simulink model "PMSM_FOC34"  (R2020b)
settings: Solver=FixedStepAuto  StartTime=0.0  StopTime=0.5  RelTol=1e-3
InitFcn:
  | Phi = 0.1;
  | Ld = 0.01;
  | Lq = 0.02;
  | Rs = 0.38;
  | p = 2;
  | Jm = 0.1e-3;
  | Dm = 1e-3;
  | Vdc = 100;
  | fc = 10e3;
  | Ts = 1/fc/100;
  | t  = 1/fc;
  | Kp_id = 3.6687;
  | Ki_id = 387.9764;
  | Kp_iq = 133.9450;
  | Ki_iq = 977.0344;
  | Kp_s = 0.0276;
  | Ki_s = 0.1598;
values from neighbouring files (symbols this model uses):
  s1 = 1    [simulink_data_collection_labelling_PMSM_CODE.m]
  s2 = 1    [simulink_data_collection_labelling_PMSM_CODE.m]
  s3 = 1    [simulink_data_collection_labelling_PMSM_CODE.m]
  s4 = 1    [simulink_data_collection_labelling_PMSM_CODE.m]
  s5 = 0    [simulink_data_collection_labelling_PMSM_CODE.m]
  s6 = 0    [simulink_data_collection_labelling_PMSM_CODE.m]
libraries: powerlib x11, fl_lib x6, nesl_utility x5, pid_lib x3, eeTransforms x2, simulink x1
settings Model: Creator=shirl  LastModifiedBy=alade
settings DataIOCC: ReturnWorkspaceOutputs=off
settings SFSimCC: CustomCodeUndefinedFunction=UseInterfaceOnly

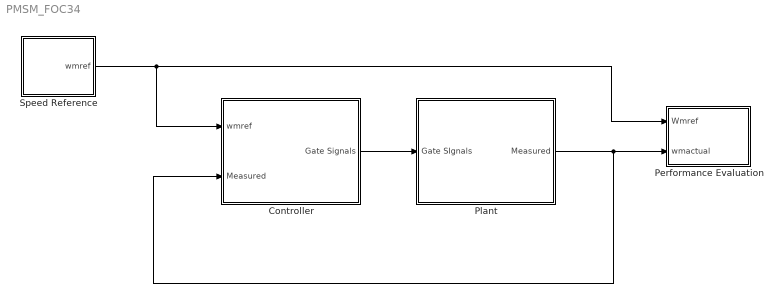
== system PMSM_FOC34 ==
  Controller : Subsystem
  Performance Evaluation : Subsystem
  Plant : Subsystem
  Speed Reference : Subsystem
  wires:
  Controller/1(Gate Signals) -> Plant/1(Gate SIgnals)
  Speed Reference/1(wmref) -> Performance Evaluation/1(Wmref), Controller/1(wmref)
  Plant/1(Measured) -> Performance Evaluation/2(wmactual), Controller/2(Measured)

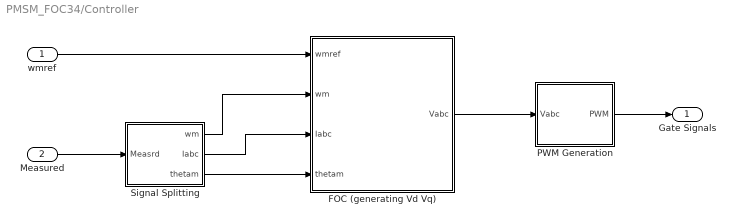
== system PMSM_FOC34/Controller ==
  wmref : Inport
  Measured : Inport  Port=2
  FOC (generating Vd Vq) : Subsystem
  PWM Generation : Subsystem
  Signal Splitting : Subsystem
  Gate Signals : Outport  VectorParamsAs1DForOutWhenUnconnected=off
  wires:
  FOC (generating Vd Vq)/1(Vabc) -> PWM Generation/1(Vabc)
  PWM Generation/1(PWM) -> Gate Signals/1
  wmref/1 -> FOC (generating Vd Vq)/1(wmref)
  Measured/1 -> Signal Splitting/1(Measrd)
  Signal Splitting/1(wm) -> FOC (generating Vd Vq)/2(wm)
  Signal Splitting/2(Iabc) -> FOC (generating Vd Vq)/3(Iabc)
  Signal Splitting/3(thetam) -> FOC (generating Vd Vq)/4(thetam)

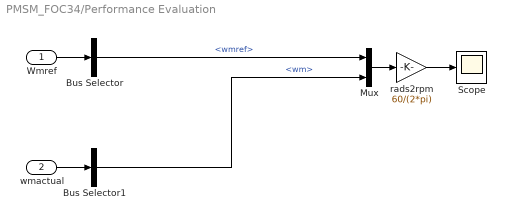
== system PMSM_FOC34/Performance Evaluation ==
  Wmref : Inport
  wmactual : Inport  Port=2
  Bus Selector : BusSelector  OutputSignals=wmref
  Bus Selector1 : BusSelector  OutputSignals=wm
  Mux : Mux  Inputs=2
  Scope : Scope
  rads2rpm : Gain  Gain=60/(2*pi)
  wires:
  Wmref/1 -> Bus Selector/1
  Mux/1 -> rads2rpm/1
  rads2rpm/1 -> Scope/1
  wmactual/1 -> Bus Selector1/1
  Bus Selector/1 -> Mux/1  "<wmref>"
  Bus Selector1/1 -> Mux/2  "<wm>"

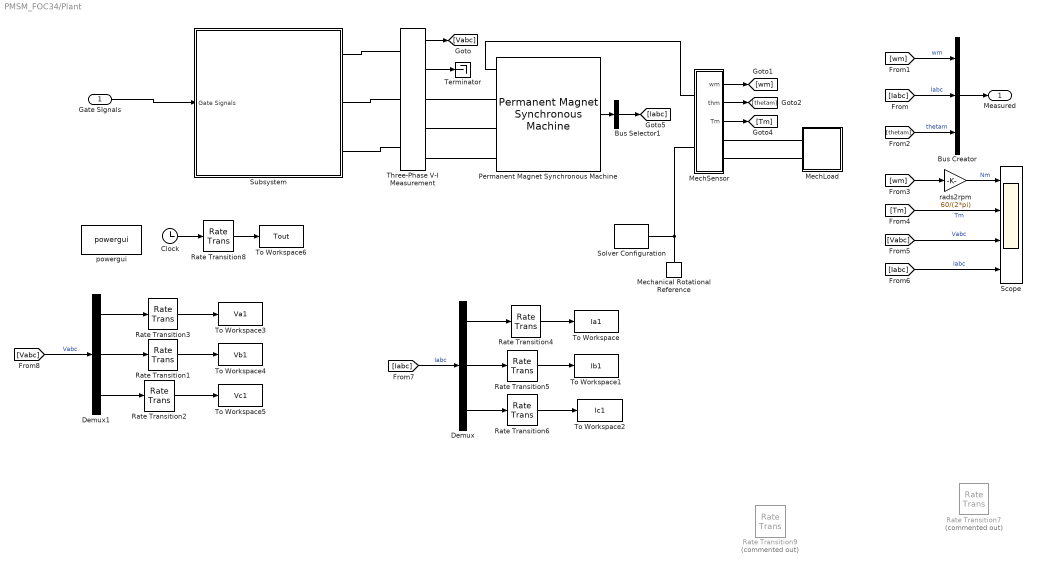
== system PMSM_FOC34/Plant ==
  Gate SIgnals : Inport
  Bus Creator : BusCreator  Inputs=3
  Bus Selector1 : BusSelector  OutputSignals=Stator current is_a (A),Stator current is_b (A),Stator current is_c (A)  OutputAsBus=on
  Clock : Clock
  Demux : Demux  Outputs=3
  Demux1 : Demux  Outputs=3
  MechLoad : Subsystem
  MechSensor : Subsystem
  Mechanical Rotational Reference : fl_lib/Mechanical/Rotational Elements/Mechanical Rotational Reference
  Permanent Magnet Synchronous Machine : powerlib/Machines/Permanent Magnet Synchronous Machine  NbPhases=3  FluxDistribution=Sinusoidal  RotorType=Salient-pole  MechanicalLoad=Mechanical rotational port  PresetModel=No  ShowDetailedParameters=on  MeasurementBus=off  Resistance=Rs  Inductance=8.5e-3  dqInductances=[Ld, Lq]  La=0.000395  MachineConstant=Flux linkage established by magnets (V.s)  Flux=Phi  VoltageCst=36.276  TorqueCst=0.3  Flat=120  Mechanical=[1e-9 0 p 0]  PolePairs=4  InitialConditions=[0,0, 0,0]  InitialConditions5ph=[0 0 0 0 0 0]  RefAngle=Aligned with phase A axis (original Park)  IterativeDiscreteModel=Trapezoidal non iterative  TsBlock=-1  TsPowergui=0
  Rate Transition{1..6,8} (7 alike) : RateTransition  OutPortSampleTime=10^-3
  Rate Transition7 : RateTransition  Commented=on  OutPortSampleTime=10^-4
  Rate Transition9 : RateTransition  Commented=on  OutPortSampleTime=10^-3
  Scope : Scope  NumInputPorts=4
  Solver Configuration : nesl_utility/Solver Configuration  PhysicalDomain=network_engine_domain  SubClassName=solver  LeftPortType=input  RightPortType=generic  Tones=[]  Harmonics=[]  SimulateNoise=off  Profile=off  UseLocalSampling=off  EnableSwitchedLinearOptims=on  FrequencyDomain=off  UseCCode=off  RelTol=0.001  AbsTol=1e-06  MinStep=1e-09  ToWorkspace=off  RevertToSquareIcSolve=off  NumHomotopyIterations=100  PhasorMode=off  PhasorModeNumHarmonics=1  DoDC=off  ResidualTolerance=1e-09  UseLocalSolver=off  LocalSolverChoice=NE_BACKWARD_EULER_ADVANCER  LocalSolverSampleTime=0.001  DoFixedCost=off  MaxNonlinIter=3  MaxModeIter=2  ComputeImpulses=off  ImpulseIterations=2  LinearAlgebra=Sparse  EquationFormulation=NE_TIME_EF  DelaysMemoryBudget=1024  AutomaticFiltering=on  FilteringTimeConstant=0.001  PartitionStorageMethod=AS_NEEDED  PartitionMemoryBudget=1024  PartitionMethod=FAST
  Subsystem : Subsystem
  Terminator : Terminator
  Three-Phase V-I Measurement : powerlib/Measurements/Three-Phase V-I Measurement  VoltageMeasurement=phase-to-phase  SetLabelV=off  LabelV=Vabc  Vpu=off  VpuLL=off  CurrentMeasurement=yes  SetLabelI=off  LabelI=Iabc  Ipu=off  Pbase=100e6  Vbase=500e3  OutputType=Complex  PhasorSimulation=off  PSBequivalent=0
  To Workspace : ToWorkspace  VariableName=Ia1  SampleTime=-1
      settings: Save2DSignal=2-D array (concatenate along first dimension)
  To Workspace1 : ToWorkspace  VariableName=Ib1  SampleTime=-1
      settings: Save2DSignal=2-D array (concatenate along first dimension)
  To Workspace2 : ToWorkspace  VariableName=Ic1  SampleTime=-1
      settings: Save2DSignal=2-D array (concatenate along first dimension)
  To Workspace3 : ToWorkspace  VariableName=Va1  SampleTime=-1
      settings: Save2DSignal=2-D array (concatenate along first dimension)
  To Workspace4 : ToWorkspace  VariableName=Vb1  SampleTime=-1
      settings: Save2DSignal=2-D array (concatenate along first dimension)
  To Workspace5 : ToWorkspace  VariableName=Vc1  SampleTime=-1
      settings: Save2DSignal=2-D array (concatenate along first dimension)
  To Workspace6 : ToWorkspace  VariableName=Tout  SampleTime=-1
      settings: Save2DSignal=2-D array (concatenate along first dimension)
  powergui : powerlib/powergui  Priority=1  SimulationMode=Discrete  SampleTime=Ts  frequency=60  Iterations=50  frequencyindice=0  Pbase=100e6  ErrMax=1e-4  UnitsV=kV  UnitsW=MW  buscounter=0  FunctionMessages=off  echomessages=off  EnableUseOfTLC=off  CurrentSourceSwitches=off  DisableSnubberDevices=off  DisableRonSwitches=off  DisableVfSwitches=off  DisplayEquations=off  AutomaticDiscreteSolvers=off  SolverType=Tustin/Backward Euler (TBE)  Interpol=off  ExternalGateDelay=off  methode=off  Ts=100  x0status=blocks  SPID=on  SwTol=0  HookPort=off  NonlinearTolerance=0  nMaxIteration=15  ContinueOnMaxIteration=off  RestoreLinks=warning  ResistiveCurrentMeasurement=off  Frange=[0:2:500]  Ylog=off  Xlog=on  ShowGrid=off  save=off  variable=ZData  structure=0  ZoomFFT=off  StartTime=0.0  cycles=1  DisplayStyle=1  fundamental=60  FreqAxis=off  MaxFrequency=1000  frequencyindicesteady=1  RmsSteady=1  display=off
  rads2rpm : Gain  Gain=60/(2*pi)
  Measured : Outport  VectorParamsAs1DForOutWhenUnconnected=off
  wires:
  MechSensor/1(wm) -> [wm]
  MechSensor/2(thm) -> [thetam]
  MechSensor/3(Tm) -> [Tm]
  [wm] -> Bus Creator/1  "wm"
  [Iabc] -> Bus Creator/2  "Iabc"
  [thetam] -> Bus Creator/3  "thetam"
  Bus Creator/1 -> Measured/1
  Gate SIgnals/1 -> Subsystem/1(Gate Signals)
  rads2rpm/1 -> Scope/1  "Nm"
  [Tm] -> Scope/2  "Tm"
  [Vabc] -> Scope/3  "Vabc"
  [Iabc] -> Scope/4  "Iabc"
  [wm] -> rads2rpm/1
  Bus Selector1/1 -> [Iabc]
  Permanent Magnet Synchronous Machine/1 -> Bus Selector1/1
  Three-Phase V-I Measurement/1 -> [Vabc]
  Three-Phase V-I Measurement/2 -> Terminator/1
  [Iabc] -> Demux/1  "Iabc"
  [Vabc] -> Demux1/1  "Vabc"
  Rate Transition1/1 -> To Workspace4/1
  Demux1/2 -> Rate Transition1/1
  Rate Transition2/1 -> To Workspace5/1
  Demux1/3 -> Rate Transition2/1
  Rate Transition8/1 -> To Workspace6/1
  Demux1/1 -> Rate Transition3/1
  Rate Transition3/1 -> To Workspace3/1
  Rate Transition4/1 -> To Workspace/1
  Rate Transition5/1 -> To Workspace1/1
  Rate Transition6/1 -> To Workspace2/1
  Demux/1 -> Rate Transition4/1
  Demux/2 -> Rate Transition5/1
  Demux/3 -> Rate Transition6/1
  Clock/1 -> Rate Transition8/1
  connections:
  Mechanical Rotational Reference/LConn1 -- MechSensor/LConn2 -- Solver Configuration/RConn1
  MechSensor/RConn1 -- MechLoad/LConn1
  MechSensor/RConn2 -- MechLoad/LConn2
  Permanent Magnet Synchronous Machine/LConn1 -- MechSensor/LConn1
  Three-Phase V-I Measurement/RConn1 -- Permanent Magnet Synchronous Machine/LConn2
  Three-Phase V-I Measurement/RConn2 -- Permanent Magnet Synchronous Machine/LConn3
  Three-Phase V-I Measurement/RConn3 -- Permanent Magnet Synchronous Machine/LConn4
  Subsystem/RConn1 -- Three-Phase V-I Measurement/LConn1
  Three-Phase V-I Measurement/LConn3 -- Subsystem/RConn3
  Three-Phase V-I Measurement/LConn2 -- Subsystem/RConn2

== system PMSM_FOC34/Speed Reference ==
  Bus Creator : BusCreator  Inputs=1
  Nmref1 : Step  Time=0  After=1000  SampleTime=0
  rpm2rads : Gain  Gain=2*pi/60
  wmref : Outport  VectorParamsAs1DForOutWhenUnconnected=off
  wires:
  rpm2rads/1 -> Bus Creator/1  "wmref"
  Bus Creator/1 -> wmref/1
  Nmref1/1 -> rpm2rads/1

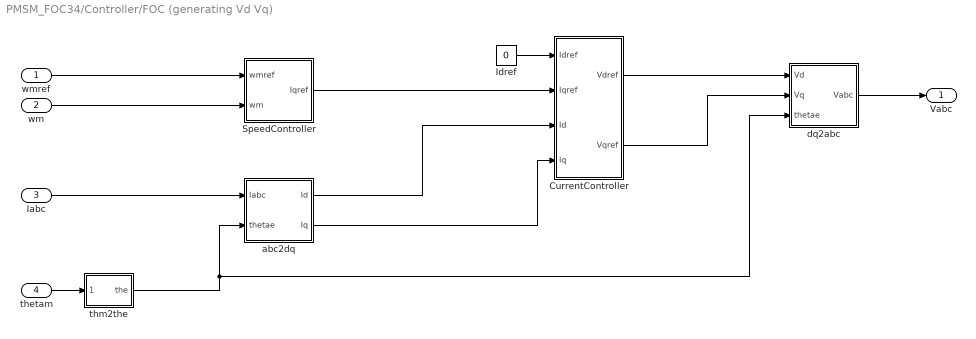
== system PMSM_FOC34/Controller/FOC (generating Vd Vq) ==
  wmref : Inport
  wm : Inport  Port=2
  Iabc : Inport  Port=3
  thetam : Inport  Port=4
  CurrentController : Subsystem
  Idref : Constant  Value=0  SampleTime=-1
  SpeedController : Subsystem
  abc2dq : Subsystem
  dq2abc : Subsystem
  thm2the : Subsystem
  Vabc : Outport  VectorParamsAs1DForOutWhenUnconnected=off
  wires:
  abc2dq/2(Iq) -> CurrentController/4(Iq)
  wmref/1 -> SpeedController/1(wmref)
  abc2dq/1(Id) -> CurrentController/3(Id)
  Iabc/1 -> abc2dq/1(Iabc)
  CurrentController/1(Vdref) -> dq2abc/1(Vd)
  CurrentController/2(Vqref) -> dq2abc/2(Vq)
  wm/1 -> SpeedController/2(wm)
  Idref/1 -> CurrentController/1(Idref)
  dq2abc/1(Vabc) -> Vabc/1
  SpeedController/1(Iqref) -> CurrentController/2(Iqref)
  thm2the/1(the) -> abc2dq/2(thetae), dq2abc/3(thetae)
  thetam/1 -> thm2the/1(thm)

== system PMSM_FOC34/Controller/PWM Generation ==
  Vabc : Inport
  Gain : Gain  Gain=1/(Vdc/2)
  Sine PWM : Subsystem
  PWM : Outport  VectorParamsAs1DForOutWhenUnconnected=off
  wires:
  Sine PWM/1(PWM) -> PWM/1
  Vabc/1 -> Gain/1  "Vabc"
  Gain/1 -> Sine PWM/1(Vs*)

== system PMSM_FOC34/Controller/Signal Splitting ==
  Measrd : Inport
  Bus Selector : BusSelector  OutputSignals=wm,Iabc,thetam
  wm : Outport  VectorParamsAs1DForOutWhenUnconnected=off
  Iabc : Outport  Port=2  VectorParamsAs1DForOutWhenUnconnected=off
  thetam : Outport  Port=3  VectorParamsAs1DForOutWhenUnconnected=off
  wires:
  Measrd/1 -> Bus Selector/1
  Bus Selector/2 -> Iabc/1  "<Iabc>"
  Bus Selector/1 -> wm/1  "<wm>"
  Bus Selector/3 -> thetam/1  "<thetam>"

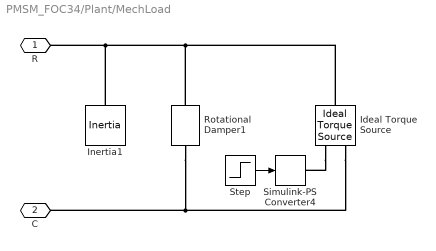
== system PMSM_FOC34/Plant/MechLoad ==
  Ideal Torque Source : fl_lib/Mechanical/Mechanical Sources/Ideal Torque Source
  Inertia1 : fl_lib/Mechanical/Rotational Elements/Inertia  inertia=Jm kg*m^2  num_ports=foundation.enum.numPorts2.one  w_specify=off  w_priority=High  w=0 rad/s  w_nominal_specify=off  w_nominal_unit=rad/s  w_nominal_value=1  t_specify=off  t_priority=None  t=0 N*m  t_nominal_specify=off  t_nominal_unit=N*m  t_nominal_value=1
  Rotational Damper1 : fl_lib/Mechanical/Rotational Elements/Rotational Damper  D=Dm N*m/(rad/s)  w_specify=off  w_priority=None  w=0 rad/s  w_nominal_specify=off  w_nominal_unit=rad/s  w_nominal_value=1  t_specify=off  t_priority=None  t=0 N*m  t_nominal_specify=off  t_nominal_unit=N*m  t_nominal_value=1
  Simulink-PS Converter4 : nesl_utility/Simulink-PS Converter  PhysicalDomain=network_engine_domain  SubClassName=ps_input  LeftPortType=input  RightPortType=output  PseudoPeriodic=off  Frequencies=[]  NoiseDistribution=none  NoiseParameters=[]  Unit=1  AffineConversion=off  FilteringAndDerivatives=provide  SimscapeFilterOrder=1  InputFilterTimeConstant=0.001  UdotUserProvided=0
  Step : Step  Time=10  After=0.2  SampleTime=0
  R : PMIOPort  Side=Left
  C : PMIOPort  Port=2  Side=Left
  wires:
  Step/1 -> Simulink-PS Converter4/1
  connections:
  Ideal Torque Source/RConn1 -- Simulink-PS Converter4/RConn1
  Ideal Torque Source/RConn2 -- Rotational Damper1/RConn1 -- C/RConn1
  Ideal Torque Source/LConn1 -- Rotational Damper1/LConn1 -- Inertia1/LConn1 -- R/RConn1

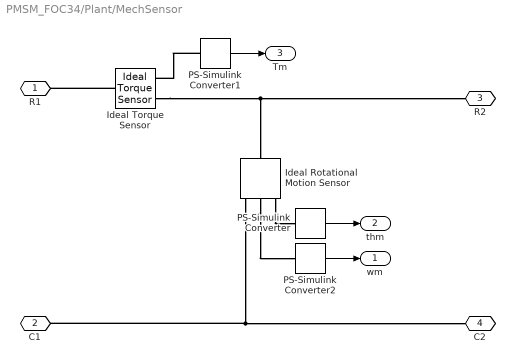
== system PMSM_FOC34/Plant/MechSensor ==
  Ideal Rotational Motion Sensor : fl_lib/Mechanical/Mechanical Sensors/Ideal Rotational Motion Sensor  wrap_angle=simscape.enum.onoff.off  offset=0 rad
  Ideal Torque Sensor : fl_lib/Mechanical/Mechanical Sensors/Ideal Torque Sensor
  PS-Simulink Converter : nesl_utility/PS-Simulink Converter  PhysicalDomain=network_engine_domain  SubClassName=ps_output  LeftPortType=input  RightPortType=output  PseudoPeriodic=off  Frequencies=[]  Unit=1  AffineConversion=off
  PS-Simulink Converter1 : nesl_utility/PS-Simulink Converter  PhysicalDomain=network_engine_domain  SubClassName=ps_output  LeftPortType=input  RightPortType=output  PseudoPeriodic=off  Frequencies=[]  Unit=1  AffineConversion=off
  PS-Simulink Converter2 : nesl_utility/PS-Simulink Converter  PhysicalDomain=network_engine_domain  SubClassName=ps_output  LeftPortType=input  RightPortType=output  PseudoPeriodic=off  Frequencies=[]  Unit=1  AffineConversion=off
  R1 : PMIOPort  Side=Left
  C1 : PMIOPort  Port=2  Side=Left
  R2 : PMIOPort  Port=3  Side=Right
  C2 : PMIOPort  Port=4  Side=Right
  wm : Outport  VectorParamsAs1DForOutWhenUnconnected=off
  thm : Outport  Port=2  VectorParamsAs1DForOutWhenUnconnected=off
  Tm : Outport  Port=3  VectorParamsAs1DForOutWhenUnconnected=off
  wires:
  PS-Simulink Converter/1 -> thm/1
  PS-Simulink Converter1/1 -> Tm/1
  PS-Simulink Converter2/1 -> wm/1
  connections:
  Ideal Rotational Motion Sensor/RConn3 -- PS-Simulink Converter/LConn1
  Ideal Rotational Motion Sensor/RConn1 -- C2/RConn1 -- C1/RConn1
  Ideal Torque Sensor/LConn1 -- R1/RConn1
  Ideal Torque Sensor/RConn1 -- R2/RConn1 -- Ideal Rotational Motion Sensor/LConn1
  PS-Simulink Converter1/LConn1 -- Ideal Torque Sensor/RConn2
  Ideal Rotational Motion Sensor/RConn2 -- PS-Simulink Converter2/LConn1

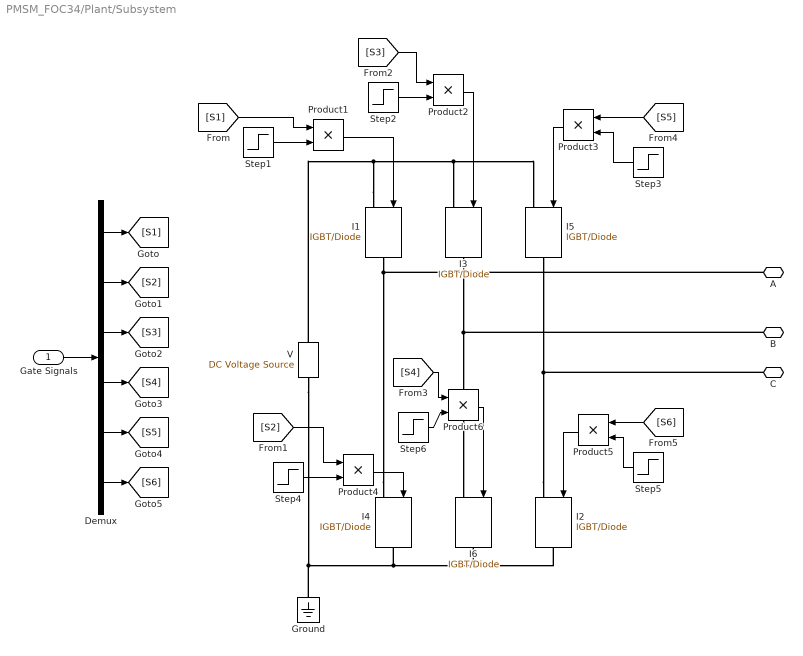
== system PMSM_FOC34/Plant/Subsystem ==
  Gate Signals : Inport
  Demux : Demux  Outputs=6
  Ground : powerlib/Elements/Ground  LConnTagsString=a
  I{1..6} (6 alike) : powerlib/Power Electronics/IGBT//Diode  Ron=1e-3  Rs=1e5  Cs=inf  Measurements=off
  Product{1..6} (6 alike) : Product
  Step1 : Step  Time=0.2  Before=1  After=s1  SampleTime=0
  Step2 : Step  Time=0.2  Before=1  After=s3  SampleTime=0
  Step3 : Step  Time=0.2  Before=1  After=s5  SampleTime=0
  Step4 : Step  Time=0.2  Before=1  After=s2  SampleTime=0
  Step5 : Step  Time=0.2  Before=1  After=s6  SampleTime=0
  Step6 : Step  Time=0.2  Before=1  After=s4  SampleTime=0
  V : powerlib/Electrical Sources/DC Voltage Source  Amplitude=Vdc  Measurements=None
  "A " : PMIOPort  Side=Right
  "B " : PMIOPort  Port=2  Side=Right
  "C " : PMIOPort  Port=3  Side=Right
  wires:
  Demux/1 -> [S1]
  Demux/4 -> [S4]
  Demux/3 -> [S3]
  Demux/2 -> [S2]
  Gate Signals/1 -> Demux/1
  Demux/5 -> [S5]
  Demux/6 -> [S6]
  Step1/1 -> Product1/2
  Step2/1 -> Product2/2
  Product1/1 -> I1/1
  [S1] -> Product1/1
  Step3/1 -> Product3/2
  Step4/1 -> Product4/2
  Step5/1 -> Product5/2
  Step6/1 -> Product6/2
  Product2/1 -> I3/1
  [S3] -> Product2/1
  Product3/1 -> I5/1
  [S5] -> Product3/1
  Product4/1 -> I4/1
  [S2] -> Product4/1
  Product6/1 -> I6/1
  [S4] -> Product6/1
  Product5/1 -> I2/1
  [S6] -> Product5/1
  connections:
  I1/LConn1 -- I5/LConn1 -- I3/LConn1 -- V/RConn1
  I4/LConn1 -- I1/RConn1 -- "A "/RConn1
  I6/RConn1 -- Ground/LConn1 -- V/LConn1 -- I4/RConn1 -- I2/RConn1
  I2/LConn1 -- "C "/RConn1 -- I5/RConn1
  I3/RConn1 -- "B "/RConn1 -- I6/LConn1

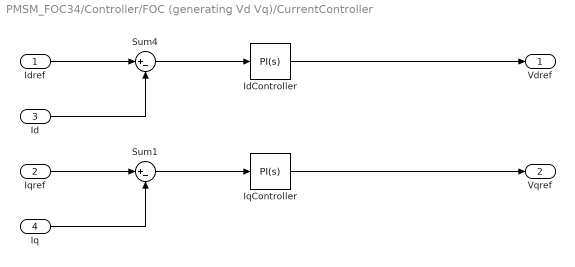
== system PMSM_FOC34/Controller/FOC (generating Vd Vq)/CurrentController ==
  Idref : Inport
  Iqref : Inport  Port=2
  Id : Inport  Port=3
  Iq : Inport  Port=4
  IdController : pid_lib/PID Controller  Controller=PI  Form=Parallel  TimeDomain=Continuous-time  UseExternalTs=off  SampleTime=-1  IntegratorMethod=Forward Euler  FilterMethod=Forward Euler  ControllerParametersSource=internal  P=Kp_id  I=Ki_id  D=0  UseFilter=on  N=100  TunerSelectOption=Transfer Function Based (PID Tuner App)  InitialConditionSource=internal  InitialConditionForIntegrator=0  InitialConditionForFilter=0  DifferentiatorICPrevScaledInput=0  ExternalReset=none  TrackingMode=off  Kt=1  LimitOutput=off  SatLimitsSource=internal  UpperSaturationLimit=inf  LowerSaturationLimit=-inf  LinearizeAsGain=on  AntiWindupMode=none  Kb=1  POutMin=[]  POutMax=[]  IOutMin=[]  IOutMax=[]  DOutMin=[]  DOutMax=[]  NOutMin=[]  NOutMax=[]  SumOutMin=[]  SumOutMax=[]  SaturationOutMin=[]  SaturationOutMax=[]  PParamMin=[]  PParamMax=[]  IParamMin=[]  IParamMax=[]  DParamMin=[]  DParamMax=[]  NParamMin=[]  NParamMax=[]  KbParamMin=[]  KbParamMax=[]  KtParamMin=[]  KtParamMax=[]  KbOutMin=[]  KbOutMax=[]  KtOutMin=[]  KtOutMax=[]  IntegratorOutMin=[]  IntegratorOutMax=[]  FilterOutMin=[]  FilterOutMax=[]  SumI1OutMin=[]  SumI1OutMax=[]  SumI2OutMin=[]  SumI2OutMax=[]  SumI3OutMin=[]  SumI3OutMax=[]  SumI4OutMin=[]  SumI4OutMax=[]  SumDOutMin=[]  SumDOutMax=[]  DifferentiatorOutMin=[]  DifferentiatorOutMax=[]  FilterDiffOutCoefMin=[]  FilterDiffOutCoefMax=[]  ReciprocalOutMin=[]  ReciprocalOutMax=[]  SumDenOutMin=[]  SumDenOutMax=[]  SumNumOutMin=[]  SumNumOutMax=[]  DivideOutMin=[]  DivideOutMax=[]  UdiffTsProdOutMin=[]  UdiffTsProdOutMax=[]  NTsProdOutMin=[]  NTsProdOutMax=[]  UintegralTsProdOutMin=[]  UintegralTsProdOutMax=[]  UngainTsProdOutMin=[]  UngainTsProdOutMax=[]  IntegratorContinuousStateAttributes=''  IntegratorStateMustResolveToSignalObject=off  IntegratorRTWStateStorageClass=Auto  FilterContinuousStateAttributes=''  FilterStateMustResolveToSignalObject=off  FilterRTWStateStorageClass=Auto  ParallelPVariant=InternalParameters  IdealPVariant=Disabled  IVariant=InternalParameters  DVariant=Disabled  IntegratorVariant=Continuous  SatVariant=Disabled  AWVariant=Passthrough  PCopyVariant=Disabled  TRVariant=Disabled  FdbkBlocksVariant=Forward  IdealPFdbkVariant=Disabled  SatFdbkVariant=Disabled  DerivativeFilterVariant=Disabled  NVariant=Disabled  NCopyVariant=Disabled_SignalSpec  FilterICVariant=Disabled  IntegratorICVariant=InternalICs  ExternalResetVariant=Disabled  TRSumVariant=Passthrough  SumFdbkVariant=Disabled  SumVariant=Sum_PI  TsampFilterVariant=InternalTs  TsampNgainVariant=Passthrough  TsampIntegralVariant=Passthrough  ExternalSaturationOutDataTypeStr=Inherit: Same as second input
  IqController : pid_lib/PID Controller  Controller=PI  Form=Parallel  TimeDomain=Continuous-time  UseExternalTs=off  SampleTime=-1  IntegratorMethod=Forward Euler  FilterMethod=Forward Euler  ControllerParametersSource=internal  P=Kp_iq  I=Ki_iq  D=0  UseFilter=on  N=100  TunerSelectOption=Transfer Function Based (PID Tuner App)  InitialConditionSource=internal  InitialConditionForIntegrator=0  InitialConditionForFilter=0  DifferentiatorICPrevScaledInput=0  ExternalReset=none  TrackingMode=off  Kt=1  LimitOutput=off  SatLimitsSource=internal  UpperSaturationLimit=inf  LowerSaturationLimit=-inf  LinearizeAsGain=on  AntiWindupMode=none  Kb=1  POutMin=[]  POutMax=[]  IOutMin=[]  IOutMax=[]  DOutMin=[]  DOutMax=[]  NOutMin=[]  NOutMax=[]  SumOutMin=[]  SumOutMax=[]  SaturationOutMin=[]  SaturationOutMax=[]  PParamMin=[]  PParamMax=[]  IParamMin=[]  IParamMax=[]  DParamMin=[]  DParamMax=[]  NParamMin=[]  NParamMax=[]  KbParamMin=[]  KbParamMax=[]  KtParamMin=[]  KtParamMax=[]  KbOutMin=[]  KbOutMax=[]  KtOutMin=[]  KtOutMax=[]  IntegratorOutMin=[]  IntegratorOutMax=[]  FilterOutMin=[]  FilterOutMax=[]  SumI1OutMin=[]  SumI1OutMax=[]  SumI2OutMin=[]  SumI2OutMax=[]  SumI3OutMin=[]  SumI3OutMax=[]  SumI4OutMin=[]  SumI4OutMax=[]  SumDOutMin=[]  SumDOutMax=[]  DifferentiatorOutMin=[]  DifferentiatorOutMax=[]  FilterDiffOutCoefMin=[]  FilterDiffOutCoefMax=[]  ReciprocalOutMin=[]  ReciprocalOutMax=[]  SumDenOutMin=[]  SumDenOutMax=[]  SumNumOutMin=[]  SumNumOutMax=[]  DivideOutMin=[]  DivideOutMax=[]  UdiffTsProdOutMin=[]  UdiffTsProdOutMax=[]  NTsProdOutMin=[]  NTsProdOutMax=[]  UintegralTsProdOutMin=[]  UintegralTsProdOutMax=[]  UngainTsProdOutMin=[]  UngainTsProdOutMax=[]  IntegratorContinuousStateAttributes=''  IntegratorStateMustResolveToSignalObject=off  IntegratorRTWStateStorageClass=Auto  FilterContinuousStateAttributes=''  FilterStateMustResolveToSignalObject=off  FilterRTWStateStorageClass=Auto  ParallelPVariant=InternalParameters  IdealPVariant=Disabled  IVariant=InternalParameters  DVariant=Disabled  IntegratorVariant=Continuous  SatVariant=Disabled  AWVariant=Passthrough  PCopyVariant=Disabled  TRVariant=Disabled  FdbkBlocksVariant=Forward  IdealPFdbkVariant=Disabled  SatFdbkVariant=Disabled  DerivativeFilterVariant=Disabled  NVariant=Disabled  NCopyVariant=Disabled_SignalSpec  FilterICVariant=Disabled  IntegratorICVariant=InternalICs  ExternalResetVariant=Disabled  TRSumVariant=Passthrough  SumFdbkVariant=Disabled  SumVariant=Sum_PI  TsampFilterVariant=InternalTs  TsampNgainVariant=Passthrough  TsampIntegralVariant=Passthrough  ExternalSaturationOutDataTypeStr=Inherit: Same as second input
  Sum1 : Sum  Inputs=|+-
  Sum4 : Sum  Inputs=|+-
  Vdref : Outport  VectorParamsAs1DForOutWhenUnconnected=off
  Vqref : Outport  Port=2  VectorParamsAs1DForOutWhenUnconnected=off
  wires:
  Idref/1 -> Sum4/1
  IdController/1 -> Vdref/1
  IqController/1 -> Vqref/1
  Iqref/1 -> Sum1/1
  Iq/1 -> Sum1/2
  Id/1 -> Sum4/2
  Sum4/1 -> IdController/1
  Sum1/1 -> IqController/1

== system PMSM_FOC34/Controller/FOC (generating Vd Vq)/SpeedController ==
  wmref : Inport
  wm : Inport  Port=2
  Gain : Gain  Gain=1/(3/2*p*Phi)
  PIDController : pid_lib/PID Controller  Controller=PI  Form=Parallel  TimeDomain=Continuous-time  UseExternalTs=off  SampleTime=-1  IntegratorMethod=Forward Euler  FilterMethod=Forward Euler  ControllerParametersSource=internal  P=Kp_s  I=Ki_s  D=0  UseFilter=on  N=100  TunerSelectOption=Transfer Function Based (PID Tuner App)  InitialConditionSource=internal  InitialConditionForIntegrator=0  InitialConditionForFilter=0  DifferentiatorICPrevScaledInput=0  ExternalReset=none  TrackingMode=off  Kt=1  LimitOutput=off  SatLimitsSource=internal  UpperSaturationLimit=inf  LowerSaturationLimit=-inf  LinearizeAsGain=on  AntiWindupMode=none  Kb=1  POutMin=[]  POutMax=[]  IOutMin=[]  IOutMax=[]  DOutMin=[]  DOutMax=[]  NOutMin=[]  NOutMax=[]  SumOutMin=[]  SumOutMax=[]  SaturationOutMin=[]  SaturationOutMax=[]  PParamMin=[]  PParamMax=[]  IParamMin=[]  IParamMax=[]  DParamMin=[]  DParamMax=[]  NParamMin=[]  NParamMax=[]  KbParamMin=[]  KbParamMax=[]  KtParamMin=[]  KtParamMax=[]  KbOutMin=[]  KbOutMax=[]  KtOutMin=[]  KtOutMax=[]  IntegratorOutMin=[]  IntegratorOutMax=[]  FilterOutMin=[]  FilterOutMax=[]  SumI1OutMin=[]  SumI1OutMax=[]  SumI2OutMin=[]  SumI2OutMax=[]  SumI3OutMin=[]  SumI3OutMax=[]  SumI4OutMin=[]  SumI4OutMax=[]  SumDOutMin=[]  SumDOutMax=[]  DifferentiatorOutMin=[]  DifferentiatorOutMax=[]  FilterDiffOutCoefMin=[]  FilterDiffOutCoefMax=[]  ReciprocalOutMin=[]  ReciprocalOutMax=[]  SumDenOutMin=[]  SumDenOutMax=[]  SumNumOutMin=[]  SumNumOutMax=[]  DivideOutMin=[]  DivideOutMax=[]  UdiffTsProdOutMin=[]  UdiffTsProdOutMax=[]  NTsProdOutMin=[]  NTsProdOutMax=[]  UintegralTsProdOutMin=[]  UintegralTsProdOutMax=[]  UngainTsProdOutMin=[]  UngainTsProdOutMax=[]  IntegratorContinuousStateAttributes=''  IntegratorStateMustResolveToSignalObject=off  IntegratorRTWStateStorageClass=Auto  FilterContinuousStateAttributes=''  FilterStateMustResolveToSignalObject=off  FilterRTWStateStorageClass=Auto  ParallelPVariant=InternalParameters  IdealPVariant=Disabled  IVariant=InternalParameters  DVariant=Disabled  IntegratorVariant=Continuous  SatVariant=Disabled  AWVariant=Passthrough  PCopyVariant=Disabled  TRVariant=Disabled  FdbkBlocksVariant=Forward  IdealPFdbkVariant=Disabled  SatFdbkVariant=Disabled  DerivativeFilterVariant=Disabled  NVariant=Disabled  NCopyVariant=Disabled_SignalSpec  FilterICVariant=Disabled  IntegratorICVariant=InternalICs  ExternalResetVariant=Disabled  TRSumVariant=Passthrough  SumFdbkVariant=Disabled  SumVariant=Sum_PI  TsampFilterVariant=InternalTs  TsampNgainVariant=Passthrough  TsampIntegralVariant=Passthrough  ExternalSaturationOutDataTypeStr=Inherit: Same as second input
  Sum : Sum  Inputs=|+-
  Iqref : Outport  VectorParamsAs1DForOutWhenUnconnected=off
  wires:
  PIDController/1 -> Gain/1
  Gain/1 -> Iqref/1
  wmref/1 -> Sum/1
  Sum/1 -> PIDController/1
  wm/1 -> Sum/2

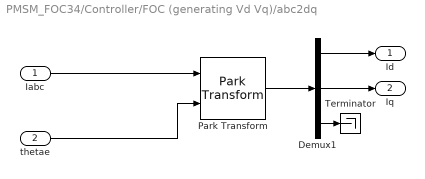
== system PMSM_FOC34/Controller/FOC (generating Vd Vq)/abc2dq ==
  Iabc : Inport
  thetae : Inport  Port=2
  Demux1 : Demux  Outputs=3
  Park Transform : eeTransforms/Park Transform  AxisAlignment=D-axis  PowerInvariant=off
  Terminator : Terminator
  Id : Outport  VectorParamsAs1DForOutWhenUnconnected=off
  Iq : Outport  Port=2  VectorParamsAs1DForOutWhenUnconnected=off
  wires:
  Iabc/1 -> Park Transform/1
  thetae/1 -> Park Transform/2
  Demux1/3 -> Terminator/1
  Park Transform/1 -> Demux1/1
  Demux1/1 -> Id/1
  Demux1/2 -> Iq/1

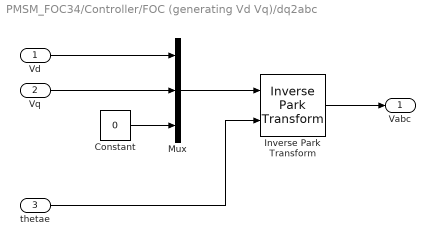
== system PMSM_FOC34/Controller/FOC (generating Vd Vq)/dq2abc ==
  Vd : Inport
  Vq : Inport  Port=2
  thetae : Inport  Port=3
  Constant : Constant  Value=0
  Inverse Park Transform : eeTransforms/Inverse Park Transform  AxisAlignment=D-axis  PowerInvariant=off
  Mux : Mux  Inputs=3
  Vabc : Outport  VectorParamsAs1DForOutWhenUnconnected=off
  wires:
  thetae/1 -> Inverse Park Transform/2
  Constant/1 -> Mux/3
  Mux/1 -> Inverse Park Transform/1
  Vd/1 -> Mux/1
  Inverse Park Transform/1 -> Vabc/1
  Vq/1 -> Mux/2

== system PMSM_FOC34/Controller/FOC (generating Vd Vq)/thm2the ==
  thm : Inport
  Constant : Constant  Value=2*pi
  Mod : Math  Operator=mod  SignedPower=on  SaturateOnIntegerOverflow=on
  PolePairs : Gain  Gain=p
  the : Outport  VectorParamsAs1DForOutWhenUnconnected=off
  wires:
  Constant/1 -> Mod/2
  PolePairs/1 -> Mod/1
  Mod/1 -> the/1
  thm/1 -> PolePairs/1

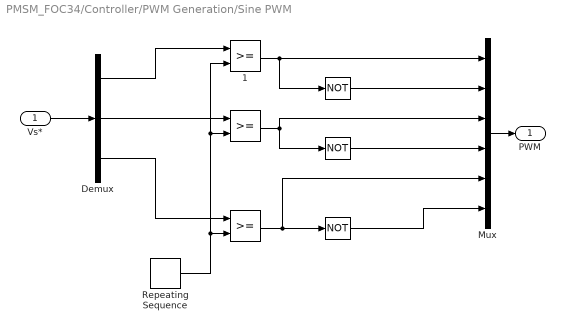
== system PMSM_FOC34/Controller/PWM Generation/Sine PWM ==
  Vs* : Inport
  "  " : RelationalOperator  OutDataTypeStr=boolean  RndMeth=Nearest
  "   " : RelationalOperator  OutDataTypeStr=boolean  RndMeth=Nearest
  "    " : Logic  Operator=NOT  AllPortsSameDT=off  OutDataTypeStr=boolean
  "     " : Logic  Operator=NOT  AllPortsSameDT=off  OutDataTypeStr=boolean
  "       " : Logic  Operator=NOT  AllPortsSameDT=off  OutDataTypeStr=boolean
  " 1" : RelationalOperator  OutDataTypeStr=boolean  RndMeth=Nearest
  Demux : Demux  Outputs=3
  Mux : Mux  Inputs=6
  Repeating Sequence : simulink/Sources/Repeating Sequence  rep_seq_t=[0 t/2 t]  rep_seq_y=[1 -1 1]
  PWM : Outport  VectorParamsAs1DForOutWhenUnconnected=off
  wires:
  Vs*/1 -> Demux/1
  Demux/1 -> " 1"/1
  Demux/2 -> "  "/1
  Demux/3 -> "   "/1
  Repeating Sequence/1 -> " 1"/2, "  "/2, "   "/2
  "       "/1 -> Mux/6
  "  "/1 -> "     "/1, Mux/3
  "   "/1 -> "       "/1, Mux/5
  "    "/1 -> Mux/2
  "     "/1 -> Mux/4
  " 1"/1 -> Mux/1, "    "/1
  Mux/1 -> PWM/1
